simulink model "emb_controller"  (R2014b)
settings: Solver=ode45  StartTime=0.0  StopTime=10  RelTol=1e-3
values from neighbouring files (symbols this model uses):
  a = [1 10501 408092434.54 2.46403599001e+12 1.14030432406e+15 22320.8207326]    [EMB_Variables.mat]
  b = 4e+12    [EMB_Variables.mat]
  c_break = 1000000    [EMB_Variables.mat]
  c_gear = 200000    [EMB_Variables.mat]
  D_Kraft = 1    [EMB_Variables.mat]
  D_Pos = 0    [EMB_Variables.mat]
  d_rot = 0.1    [EMB_Variables.mat]
  d_trans = 0.1    [EMB_Variables.mat]
  i = 113.116658706    [EMB_Variables.mat]
  I_Kraft = 1000000    [EMB_Variables.mat]
  I_Pos = 1000    [EMB_Variables.mat]
  J = 1e-05    [EMB_Variables.mat]
  K = 0.02    [EMB_Variables.mat]
  L = 0.001    [EMB_Variables.mat]
  m = 0.1    [EMB_Variables.mat]
  P_Kraft = 70000    [EMB_Variables.mat]
  P_Pos = 10000    [EMB_Variables.mat]
  R = 0.5    [EMB_Variables.mat]
  t1 = 0.0025    [EMB_Variables.mat]
  x0 = 0.05    [EMB_Variables.mat]
undefined symbols (not defined in the file or in its folder): bPC, EPSILON_R, EPSILON_T, EPSILON_W, POSITION_R, POSITION_T, sPC
libraries: simulink x4
settings Model: Creator=thomasst  LastModifiedBy=oej2si
settings DataIOCC: LimitDataPoints=off  SignalLoggingSaveFormat=ModelDataLogs
settings DebuggingCC: MultiTaskDSMMsg=warning  MultiTaskCondExecSysMsg=none
settings RTWCC: IncludeERTFirstTime=on

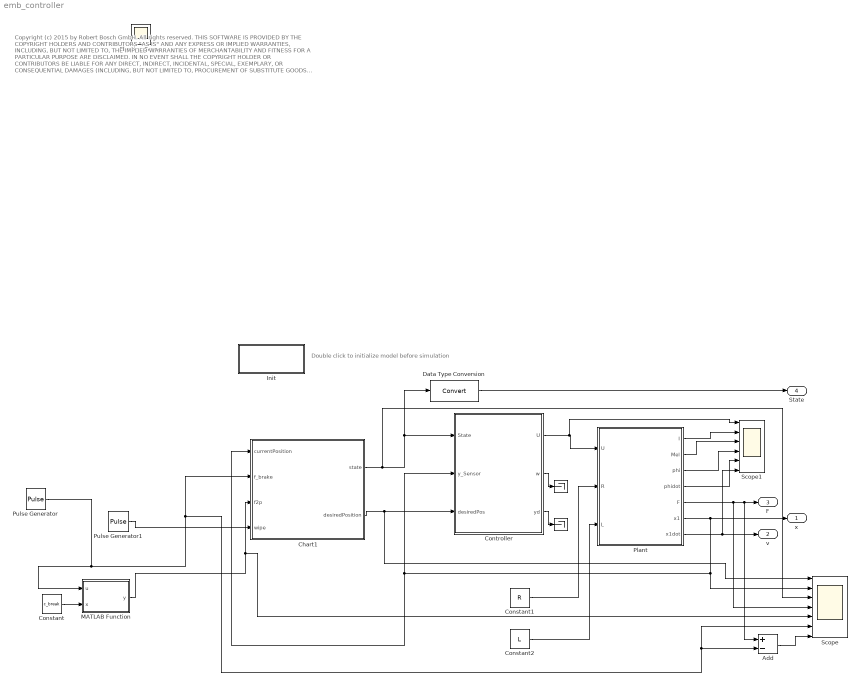
== system emb_controller ==
  note: Copyright (c) 2015 by Robert Bosch GmbH. All rights reserved.
      |
      | THIS SOFTWARE IS PROVIDED BY THE COPYRIGHT HOLDERS AND CONTRIBUTORS "AS IS"
      | AND ANY EXPRESS OR IMPLIED WARRANTIES, INCLUDING, BUT NOT LIMITED TO, THE IMPLIED
      | WARRANTIES OF MERCHANTABILITY AND FITNESS FOR A PARTICULAR PURPOSE ARE
      | DISCLAIMED. IN NO EVENT SHALL THE COPYRIGHT HOLDER OR CONTRIBUTORS BE LIABLE FOR
      | ANY DIRECT, INDIRECT, INCIDENTAL, SPECIAL, EXEMPLARY, OR CONSEQUENTIAL DAMAGES
      | (INCLUDING, BUT NOT LIMITED TO, PROCUREMENT OF SUBSTITUTE GOODS OR SERVICES;
      | LOSS OF USE, DATA, OR PROFITS; OR BUSINESS INTERRUPTION) HOWEVER CAUSED AND
      | ON ANY THEORY OF LIABILITY, WHETHER IN CONTRACT, STRICT LIABILITY, OR TORT (INCLUDING
      | NEGLIGENCE OR OTHERWISE) ARISING IN ANY WAY OUT OF THE USE OF THIS SOFTWARE, EVEN
      | IF ADVISED OF THE POSSIBILITY OF SUCH DAMAGE.
      |
      | THE ENTIRE RISK AS TO THE QUALITY AND PERFORMANCE OF THE PROGRAM IS WITH YOU. SHOULD THE PROGRAM PROVE DEFECTIVE,
      | YOU ASSUME THE COST OF ALL NECESSARY SERVICING, REPAIR OR CORRECTION.
      |
      | This is not a model of a Bosch product.
      | This model was originally released in the scope of the ARCH workshop (http://cps-vo.org/group/ARCH).
  note: Double click to initialize model before simulation
  "        " : Terminator
  "          " : Terminator
  Add : Sum  Inputs=+-
  Chart1 : Stateflow chart  TreatAsAtomicUnit=on
  Constant : Constant  Value=c_break
  Constant1 : Constant  Value=R
  Constant2 : Constant  Value=L
  Controller : Subsystem
  Data Type Conversion : DataTypeConversion
  Init : Subsystem
      settings: OpenFcn=|
      | load('EMB_Variables.mat');
      | run('EMB_Initialize');
      | run('initConstants');
  MATLAB Function : MATLAB Function  TreatAsAtomicUnit=on
  Plant : Subsystem
  Pulse Generator : DiscretePulseGenerator  PulseType=Time based  Amplitude=500  Period=0.3  PulseWidth=50  PhaseDelay=0.15
  Pulse Generator1 : DiscretePulseGenerator  PulseType=Time based  Amplitude=50  PulseWidth=50  PhaseDelay=0.15
  Scope : Scope  NumInputPorts=7
      settings: YMin=-0.01~-0.01~0~0~0~0~-600  YMax=0.06~0.06~1~600~0.0006~500~600
  Scope1 : Scope  NumInputPorts=6
      settings: YMin=-1000~-1000~-20~-1~-200~-2  YMax=1500~2500~50~5~500~5  SaveName=ScopeData5
  x : Outport
  v : Outport  Port=2
  F : Outport  Port=3
  State : Outport  Port=4
  Floating Scope : Scope
  wires:
  Plant/3(phi) -> Scope1/4
  Plant/4(phidot) -> Scope1/5
  Plant/5(F) -> Scope/4, Add/1, F/1
  Plant/7(x1dot) -> Scope1/6, v/1
  Plant/2(Mel) -> Scope1/3
  Plant/1(I) -> Scope1/2
  Plant/6(x1) -> Scope/2, Controller/2(y_Sensor), Chart1/1(currentPosition), x/1
  Controller/1(U) -> Scope1/1, Plant/1(U)
  Controller/2(w) -> "          "/1
  Controller/3(yd) -> "        "/1
  Data Type Conversion/1 -> State/1
  Constant1/1 -> Plant/2(R)
  Constant2/1 -> Plant/3(L)
  Chart1/1(state) -> Scope/3, Data Type Conversion/1, Controller/1(State)
  Chart1/2(desiredPosition) -> Scope/1, Controller/3(desiredPos)
  MATLAB Function/1(y) -> Scope/5, Chart1/3(f2p)
  Constant/1 -> MATLAB Function/2(x)
  Pulse Generator/1 -> MATLAB Function/1(u), Add/2, Scope/6, Chart1/2(f_brake)
  Pulse Generator1/1 -> Chart1/4(wipe)
  Add/1 -> Scope/7

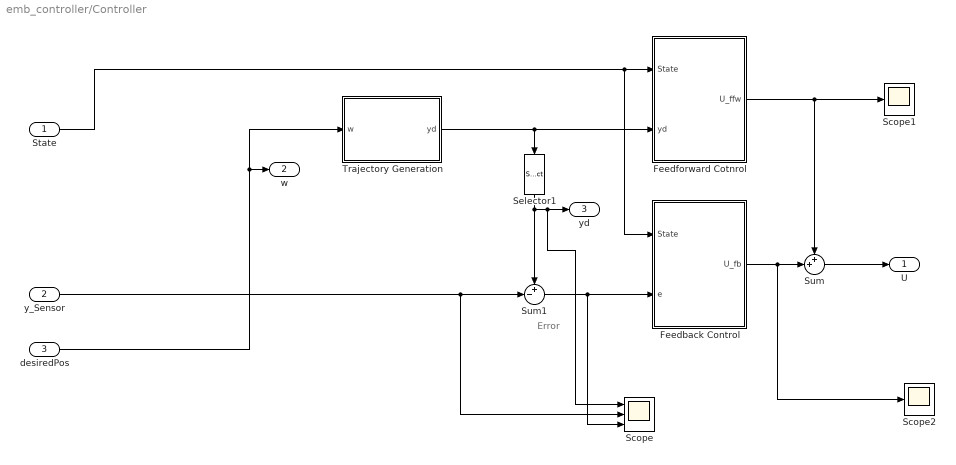
== system emb_controller/Controller ==
  note: Error
  State : Inport
  y_Sensor : Inport  Port=2
  desiredPos : Inport  Port=3
  Feedback Control : Subsystem
  Feedforward Cotnrol : Subsystem
  Scope : Scope  NumInputPorts=3
      settings: YMin=-0.1~-0.01~-0.1  YMax=1.1~0.15~1  SaveName=ScopeData2
  Scope1 : Scope
      settings: YMin=-200  YMax=1400  SaveName=ScopeData3
  Scope2 : Scope
      settings: YMin=-12000  YMax=4000  SaveName=ScopeData4
  Selector1 : Selector  InputPortWidth=6  Indices=[1]
  Sum : Sum  Inputs=++|
  Sum1 : Sum  Inputs=+-|
  Trajectory Generation : Subsystem
  U : Outport
  w : Outport  Port=2
  yd : Outport  Port=3
  wires:
  State/1 -> Feedforward Cotnrol/1(State), Feedback Control/1(State)
  desiredPos/1 -> Trajectory Generation/1(w), w/1
  Trajectory Generation/1(yd) -> Feedforward Cotnrol/2(yd), Selector1/1
  Feedforward Cotnrol/1(U_ffw) -> Sum/1, Scope1/1
  Sum/1 -> U/1
  Sum1/1 -> Scope/3, Feedback Control/2(e)
  Selector1/1 -> Sum1/1, Scope/1, yd/1
  y_Sensor/1 -> Scope/2, Sum1/2
  Feedback Control/1(U_fb) -> Scope2/1, Sum/2

== system emb_controller/Init ==

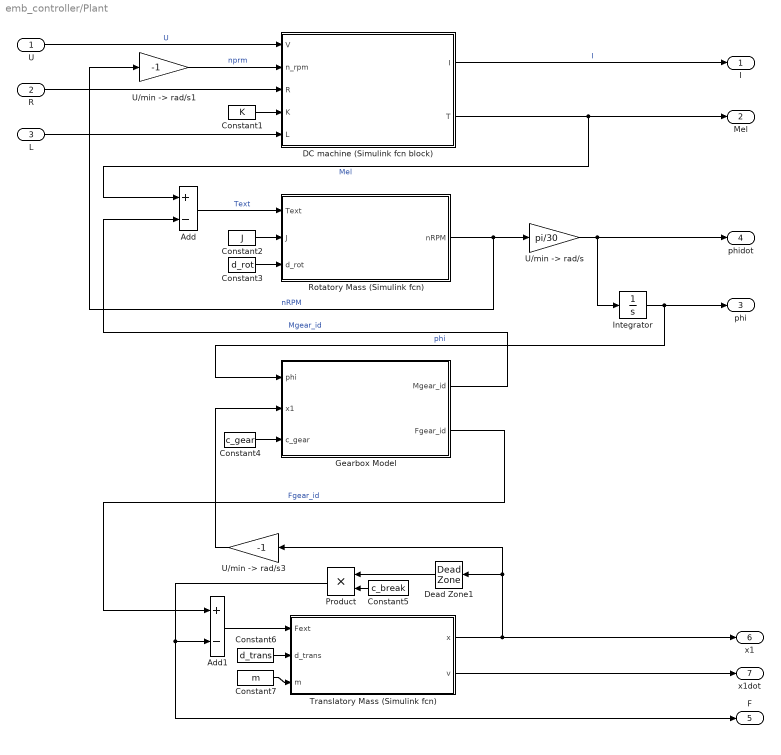
== system emb_controller/Plant ==
  U : Inport
  R : Inport  Port=2
  L : Inport  Port=3
  Add : Sum  Inputs=+-
  Add1 : Sum  Inputs=+-
  Constant1 : Constant  Value=K
  Constant2 : Constant  Value=J
  Constant3 : Constant  Value=d_rot
  Constant4 : Constant  Value=c_gear
  Constant5 : Constant  Value=c_break
  Constant6 : Constant  Value=d_trans
  Constant7 : Constant  Value=m
  DC machine (Simulink fcn block) : Subsystem
  Dead Zone1 : DeadZone  LowerValue=-inf  UpperValue=x0  SaturateOnIntegerOverflow=on
  Gearbox Model : Subsystem
  Integrator : Integrator
  Product : Product
  Rotatory Mass (Simulink fcn) : Subsystem
  Translatory Mass (Simulink fcn) : Subsystem
  "U/min -> rad/s" : Gain  Gain=pi/30
  "U/min -> rad/s1" : Gain  Gain=-1
  "U/min -> rad/s3" : Gain  Gain=-1
  I : Outport
  Mel : Outport  Port=2
  phi : Outport  Port=3
  phidot : Outport  Port=4
  F : Outport  Port=5
  x1 : Outport  Port=6
  x1dot : Outport  Port=7
  wires:
  U/1 -> DC machine (Simulink fcn block)/1(V)  "U"
  "U/min -> rad/s1"/1 -> DC machine (Simulink fcn block)/2(n_rpm)  "nprm"
  Product/1 -> F/1, Add1/2
  Dead Zone1/1 -> Product/1
  "U/min -> rad/s3"/1 -> Gearbox Model/2(x1)
  Gearbox Model/2(Fgear_id) -> Add1/1  "Fgear_id"
  Gearbox Model/1(Mgear_id) -> Add/2  "Mgear_id"
  DC machine (Simulink fcn block)/2(T) -> Mel/1, Add/1  "Mel"
  Translatory Mass (Simulink fcn)/1(x) -> Dead Zone1/1, "U/min -> rad/s3"/1, x1/1
  Add1/1 -> Translatory Mass (Simulink fcn)/1(Fext)
  Integrator/1 -> phi/1, Gearbox Model/1(phi)  "phi"
  "U/min -> rad/s"/1 -> Integrator/1, phidot/1
  Rotatory Mass (Simulink fcn)/1(nRPM) -> "U/min -> rad/s"/1, "U/min -> rad/s1"/1  "nRPM"
  Add/1 -> Rotatory Mass (Simulink fcn)/1(Text)  "Text"
  DC machine (Simulink fcn block)/1(I) -> I/1  "I"
  Translatory Mass (Simulink fcn)/2(v) -> x1dot/1
  R/1 -> DC machine (Simulink fcn block)/3(R)
  Constant1/1 -> DC machine (Simulink fcn block)/4(K)
  L/1 -> DC machine (Simulink fcn block)/5(L)
  Constant2/1 -> Rotatory Mass (Simulink fcn)/2(J)
  Constant3/1 -> Rotatory Mass (Simulink fcn)/3(d_rot)
  Constant4/1 -> Gearbox Model/3(c_gear)
  Constant5/1 -> Product/2
  Constant6/1 -> Translatory Mass (Simulink fcn)/2(d_trans)
  Constant7/1 -> Translatory Mass (Simulink fcn)/3(m)

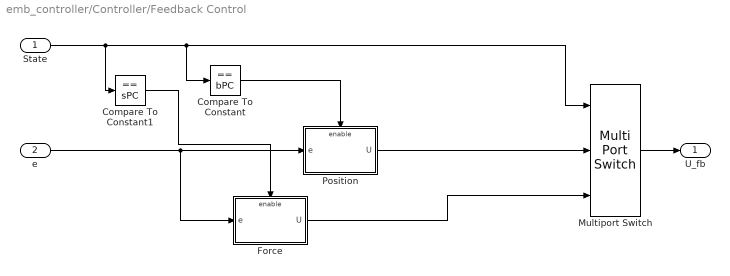
== system emb_controller/Controller/Feedback Control ==
  State : Inport
  e : Inport  Port=2
  Compare To Constant : simulink/Logic and Bit Operations/Compare To Constant  relop===  const=bPC  OutDataTypeStr=boolean
  Compare To Constant1 : simulink/Logic and Bit Operations/Compare To Constant  relop===  const=sPC  OutDataTypeStr=boolean
  Force : Subsystem  TreatAsAtomicUnit=on
  Multiport Switch : MultiPortSwitch  DataPortOrder=Zero-based contiguous  Inputs=2  zeroidx=on
  Position : Subsystem  TreatAsAtomicUnit=on
  U_fb : Outport
  wires:
  State/1 -> Compare To Constant1/1, Compare To Constant/1, Multiport Switch/1
  e/1 -> Position/1(e), Force/1(e)
  Position/1(U) -> Multiport Switch/2
  Multiport Switch/1 -> U_fb/1
  Force/1(U) -> Multiport Switch/3
  Compare To Constant/1 -> Position/Enable
  Compare To Constant1/1 -> Force/Enable

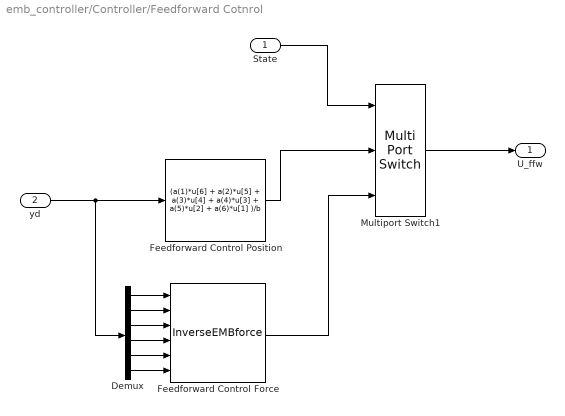
== system emb_controller/Controller/Feedforward Cotnrol ==
  State : Inport
  yd : Inport  Port=2
  Demux : Demux  Outputs=6
  Feedforward Control Force : S-Function  FunctionName=InverseEMBforce  Parameters=R,L,K,J,dvrot,m,dvtrans,cgear,i,cbreak,x0,xic  EnableBusSupport=off  mask{R=R, L=L, K=K, J=J, dvrot=d_rot, m=m, dvtrans=d_trans, cgear=c_gear, i=i, cbreak=c_break, x0=x0, xic=[0]}
      mask prompts: R "Widerstand R [Ohm]:"; L "Induktivitaet L [H]:"; K "Motorkonstante K [Vs]:"; J "Traegheitsmoment J [kgm^2]:"; dvrot "Viskose Reibung dvrot [Nms/rad]:"; m "Masse m [kg]:"; dvtrans "Viskose Reibung dvtrans [Ns/m]:"; cgear "Steifigkeit Getriebe cgear [N/m]:"; i "Uebersetzung i [-]:"; cbreak "Steifigkeit Bremse cbreak [N/m]:"; x0 "Position x0 [m]:"; xic "Vector of continuous initial conditions [Initial Dummy]"
  Feedforward Control Position : Fcn  Expr="(a(1)*u[6] + a(2)*u[5] + a(3)*u[4] + a(4)*u[3]  + a(5)*u[2] + a(6)*u[1] )/b"
  Multiport Switch1 : MultiPortSwitch  DataPortOrder=Zero-based contiguous  Inputs=2  zeroidx=on
  U_ffw : Outport
  wires:
  State/1 -> Multiport Switch1/1
  yd/1 -> Feedforward Control Position/1, Demux/1
  Demux/1 -> Feedforward Control Force/1
  Demux/2 -> Feedforward Control Force/2
  Demux/3 -> Feedforward Control Force/3
  Demux/4 -> Feedforward Control Force/4
  Demux/5 -> Feedforward Control Force/5
  Demux/6 -> Feedforward Control Force/6
  Feedforward Control Position/1 -> Multiport Switch1/2
  Feedforward Control Force/1 -> Multiport Switch1/3
  Multiport Switch1/1 -> U_ffw/1

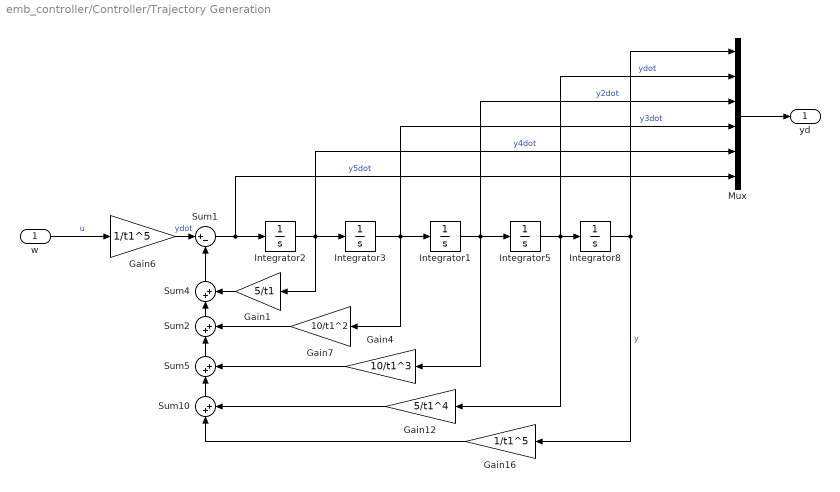
== system emb_controller/Controller/Trajectory Generation ==
  w : Inport
  Gain1 : Gain  Gain=5/t1
  Gain12 : Gain  Gain=5/t1^4
  Gain16 : Gain  Gain=1/t1^5
  Gain4 : Gain  Gain=10/t1^3
  Gain6 : Gain  Gain=1/t1^5
  Gain7 : Gain  Gain=10/t1^2
  Integrator{1..3,5,8} (5 alike) : Integrator
  Mux : Mux  Inputs=6
  Sum1 : Sum  Inputs=|+-
  Sum{2,4..5,10} (4 alike) : Sum  Inputs=|++
  yd : Outport
  wires:
  w/1 -> Gain6/1  "u"
  Mux/1 -> yd/1
  Integrator2/1 -> Gain1/1, Mux/5, Integrator3/1  "y4dot"
  Sum1/1 -> Integrator2/1, Mux/6  "y5dot"
  Gain6/1 -> Sum1/1  "ydot"
  Integrator3/1 -> Gain7/1, Mux/4, Integrator1/1  "y3dot"
  Gain7/1 -> Sum2/2
  Integrator1/1 -> Gain4/1, Mux/3, Integrator5/1  "y2dot"
  Gain4/1 -> Sum5/2
  Sum4/1 -> Sum1/2
  Gain1/1 -> Sum4/2
  Sum2/1 -> Sum4/1
  Integrator5/1 -> Gain12/1, Mux/2, Integrator8/1  "ydot"
  Sum5/1 -> Sum2/1
  Integrator8/1 -> Gain16/1, Mux/1  "y"
  Gain12/1 -> Sum10/2
  Sum10/1 -> Sum5/1
  Gain16/1 -> Sum10/1

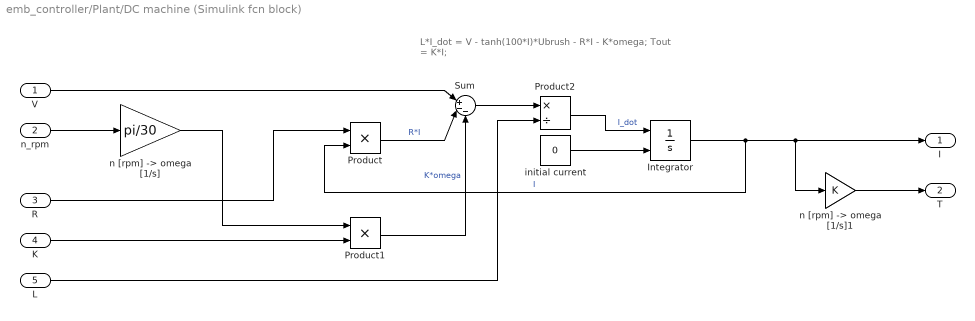
== system emb_controller/Plant/DC machine (Simulink fcn block) ==
  note: L*I_dot = V - tanh(100*I)*Ubrush - R*I - K*omega;
      | Tout = K*I;
  V : Inport
  n_rpm : Inport  Port=2
  R : Inport  Port=3
  K : Inport  Port=4
  L : Inport  Port=5
  Integrator : Integrator  InitialConditionSource=external
  Product : Product
  Product1 : Product
  Product2 : Product  Inputs=*/
  Sum : Sum  Inputs=|+--
  initial current : Constant  Value=0
  "n [rpm] -> omega [1/s]" : Gain  Gain=pi/30
  "n [rpm] -> omega [1/s]1" : Gain  Gain=K
  I : Outport
  T : Outport  Port=2
  wires:
  n_rpm/1 -> "n [rpm] -> omega [1/s]"/1
  V/1 -> Sum/1
  "n [rpm] -> omega [1/s]"/1 -> Product1/1
  Product2/1 -> Integrator/1  "I_dot"
  Integrator/1 -> Product/2, I/1, "n [rpm] -> omega [1/s]1"/1  "I"
  initial current/1 -> Integrator/2
  Product/1 -> Sum/2  "R*I"
  Product1/1 -> Sum/3  "K*omega"
  K/1 -> Product1/2
  Sum/1 -> Product2/1
  L/1 -> Product2/2
  R/1 -> Product/1
  "n [rpm] -> omega [1/s]1"/1 -> T/1

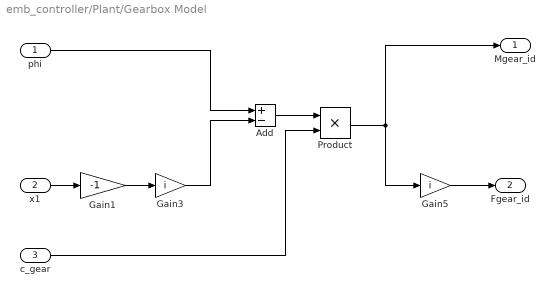
== system emb_controller/Plant/Gearbox Model ==
  phi : Inport
  x1 : Inport  Port=2
  c_gear : Inport  Port=3
  Add : Sum  Inputs=+-
  Gain1 : Gain  Gain=-1
  Gain3 : Gain  Gain=i
  Gain5 : Gain  Gain=i
  Product : Product
  Mgear_id : Outport
  Fgear_id : Outport  Port=2
  wires:
  Gain1/1 -> Gain3/1
  x1/1 -> Gain1/1
  Gain5/1 -> Fgear_id/1
  Product/1 -> Mgear_id/1, Gain5/1
  Add/1 -> Product/1
  Gain3/1 -> Add/2
  phi/1 -> Add/1
  c_gear/1 -> Product/2

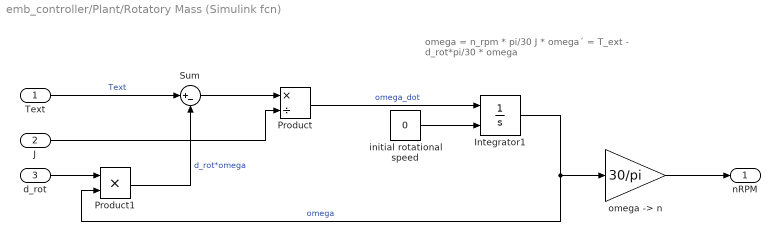
== system emb_controller/Plant/Rotatory Mass (Simulink fcn) ==
  note: omega = n_rpm * pi/30
      |
      | J * omega´ = T_ext -  d_rot*pi/30 * omega
  Text : Inport
  J : Inport  Port=2
  d_rot : Inport  Port=3
  Integrator1 : Integrator  InitialConditionSource=external
  Product : Product  Inputs=*/
  Product1 : Product
  Sum : Sum  Inputs=|+-
  initial rotational speed : Constant  Value=0
  "omega -> n " : Gain  Gain=30/pi
  nRPM : Outport
  wires:
  "omega -> n "/1 -> nRPM/1
  Product/1 -> Integrator1/1  "omega_dot"
  initial rotational speed/1 -> Integrator1/2
  Integrator1/1 -> Product1/2, "omega -> n "/1  "omega"
  Product1/1 -> Sum/2  "d_rot*omega"
  Text/1 -> Sum/1  "Text"
  d_rot/1 -> Product1/1
  Sum/1 -> Product/1
  J/1 -> Product/2

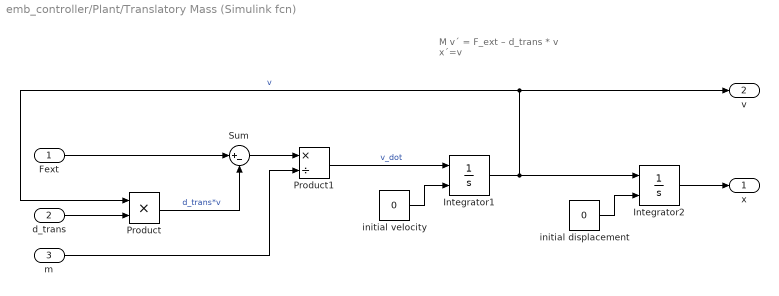
== system emb_controller/Plant/Translatory Mass (Simulink fcn) ==
  note: M v´ = F_ext – d_trans * v
      |
      | x´=v
  Fext : Inport
  d_trans : Inport  Port=2
  m : Inport  Port=3
  Integrator1 : Integrator  InitialConditionSource=external
  Integrator2 : Integrator  InitialConditionSource=external
  Product : Product
  Product1 : Product  Inputs=*/
  Sum : Sum  Inputs=|+-
  initial displacement : Constant  Value=0
  "initial velocity " : Constant  Value=0
  x : Outport
  v : Outport  Port=2
  wires:
  initial displacement/1 -> Integrator2/2
  Fext/1 -> Sum/1
  Integrator1/1 -> v/1, Product/1, Integrator2/1  "v"
  "initial velocity "/1 -> Integrator1/2
  Product1/1 -> Integrator1/1  "v_dot"
  Integrator2/1 -> x/1
  d_trans/1 -> Product/2
  Product/1 -> Sum/2  "d_trans*v"
  Sum/1 -> Product1/1
  m/1 -> Product1/2

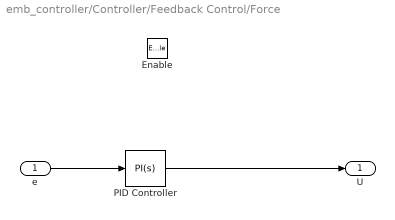
== system emb_controller/Controller/Feedback Control/Force ==
  e : Inport
  Enable : EnablePort  StatesWhenEnabling=reset
  PID Controller : simulink/Continuous/PID Controller  Controller=PI  TimeDomain=Continuous-time  SampleTime=-1  IntegratorMethod=Forward Euler  FilterMethod=Forward Euler  Form=Parallel  P=P_Kraft  I=I_Kraft  D=D_Kraft  N=100  InitialConditionSource=internal  InitialConditionForIntegrator=0  InitialConditionForFilter=0  ExternalReset=none  LimitOutput=off  UpperSaturationLimit=inf  LowerSaturationLimit=-inf  LinearizeAsGain=on  AntiWindupMode=none  Kb=1  TrackingMode=off  Kt=1  PParamMin=[]  PParamMax=[]  IParamMin=[]  IParamMax=[]  DParamMin=[]  DParamMax=[]  NParamMin=[]  NParamMax=[]  KbParamMin=[]  KbParamMax=[]  KtParamMin=[]  KtParamMax=[]  POutMin=[]  POutMax=[]  IOutMin=[]  IOutMax=[]  DOutMin=[]  DOutMax=[]  NOutMin=[]  NOutMax=[]  KbOutMin=[]  KbOutMax=[]  KtOutMin=[]  KtOutMax=[]  IntegratorOutMin=[]  IntegratorOutMax=[]  FilterOutMin=[]  FilterOutMax=[]  SumOutMin=[]  SumOutMax=[]  SumI1OutMin=[]  SumI1OutMax=[]  SumI2OutMin=[]  SumI2OutMax=[]  SumI3OutMin=[]  SumI3OutMax=[]  SumDOutMin=[]  SumDOutMax=[]  SaturationOutMin=[]  SaturationOutMax=[]  IntegratorContinuousStateAttributes=''  IntegratorStateMustResolveToSignalObject=off  IntegratorRTWStateStorageClass=Auto  FilterContinuousStateAttributes=''  FilterStateMustResolveToSignalObject=off  FilterRTWStateStorageClass=Auto  DifferentiatorICPrevScaledInput=0  DifferentiatorOutMin=[]  DifferentiatorOutMax=[]  UseFilter=on
  U : Outport
  wires:
  PID Controller/1 -> U/1
  e/1 -> PID Controller/1

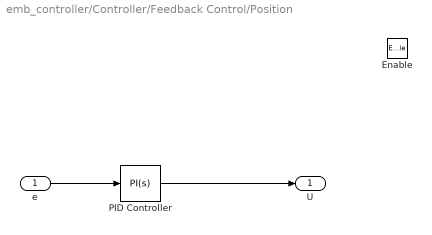
== system emb_controller/Controller/Feedback Control/Position ==
  e : Inport
  Enable : EnablePort  StatesWhenEnabling=reset
  PID Controller : simulink/Continuous/PID Controller  Controller=PI  TimeDomain=Continuous-time  SampleTime=-1  IntegratorMethod=Forward Euler  FilterMethod=Forward Euler  Form=Parallel  P=P_Pos  I=I_Pos  D=D_Pos  N=100  InitialConditionSource=internal  InitialConditionForIntegrator=0  InitialConditionForFilter=0  ExternalReset=none  LimitOutput=off  UpperSaturationLimit=inf  LowerSaturationLimit=-inf  LinearizeAsGain=on  AntiWindupMode=none  Kb=1  TrackingMode=off  Kt=1  PParamMin=[]  PParamMax=[]  IParamMin=[]  IParamMax=[]  DParamMin=[]  DParamMax=[]  NParamMin=[]  NParamMax=[]  KbParamMin=[]  KbParamMax=[]  KtParamMin=[]  KtParamMax=[]  POutMin=[]  POutMax=[]  IOutMin=[]  IOutMax=[]  DOutMin=[]  DOutMax=[]  NOutMin=[]  NOutMax=[]  KbOutMin=[]  KbOutMax=[]  KtOutMin=[]  KtOutMax=[]  IntegratorOutMin=[]  IntegratorOutMax=[]  FilterOutMin=[]  FilterOutMax=[]  SumOutMin=[]  SumOutMax=[]  SumI1OutMin=[]  SumI1OutMax=[]  SumI2OutMin=[]  SumI2OutMax=[]  SumI3OutMin=[]  SumI3OutMax=[]  SumDOutMin=[]  SumDOutMax=[]  SaturationOutMin=[]  SaturationOutMax=[]  IntegratorContinuousStateAttributes=''  IntegratorStateMustResolveToSignalObject=off  IntegratorRTWStateStorageClass=Auto  FilterContinuousStateAttributes=''  FilterStateMustResolveToSignalObject=off  FilterRTWStateStorageClass=Auto  DifferentiatorICPrevScaledInput=0  DifferentiatorOutMin=[]  DifferentiatorOutMax=[]  UseFilter=on
  U : Outport
  wires:
  e/1 -> PID Controller/1
  PID Controller/1 -> U/1

== matlab function emb_controller/MATLAB Function ==
  data: u input; y output; x input
function y = fcn(u,x)
%#codegen

y = u/x;

== stateflow chart emb_controller/Chart1 ==
  state ControllerStateCalculation [parallel]
    settings: executionOrder=2
    state bigPositionControl
      entry: state = bPC;
    state smallPositionControl
      entry: state = sPC;
    (default) -> bigPositionControl
    bigPositionControl -> smallPositionControl : [currentPosition >= POSITION_T - EPSILON_T]
    smallPositionControl -> bigPositionControl : [currentPosition < POSITION_T - EPSILON_T]
  state SetPointCalculation [parallel]
    settings: executionOrder=1
    state NotBraking
      state RestPosition
        entry: desiredPosition = POSITION_R - EPSILON_R;
        during: desiredPosition = POSITION_R - EPSILON_R;
      state Wiping
        state WipePositionContact
          entry: desiredPosition = POSITION_T + EPSILON_W;
          during: desiredPosition = POSITION_T + EPSILON_W;
        state WipePositionNoContact
          entry: desiredPosition = POSITION_T - EPSILON_W;
          during: desiredPosition = POSITION_T - EPSILON_W;
        (default) -> WipePositionContact
        WipePositionContact -> WipePositionNoContact : [currentPosition > POSITION_T]
        WipePositionNoContact -> WipePositionContact : [currentPosition <= POSITION_T]
      (default) -> RestPosition [order 1] : [wipe<=0]
      RestPosition -> Wiping : [wipe > 0]
      Wiping -> RestPosition : [wipe <= 0]
      (default) -> Wiping [order 2] : [wipe>0]
    state TouchPosition
      entry: desiredPosition = POSITION_T + f2p;
      during: desiredPosition = POSITION_T + f2p;
    (default) -> NotBraking
    NotBraking -> TouchPosition : [f_brake >0]
    TouchPosition -> NotBraking : [f_brake <= 0]
  data: state output double; currentPosition input; desiredPosition output double; f_brake input; f2p input; EPSILON_T parameter; EPSILON_R parameter; POSITION_T parameter; bPC parameter; sPC parameter; POSITION_R parameter; wipe input; EPSILON_W parameter
